simulink model "TST_EISGov_SelectParameter"  (R2016b)
settings: Solver=FixedStepDiscrete  StartTime=0.0  StopTime=simTime  FixedStep=sampleTime  RelTol=1e-3
values from neighbouring files (symbols this model uses):
  testCase = 1    [initTST_EISGov_SelectParameter_001.m]
libraries: simulink x26, UnitTest_Lib x24
(part 2 of 3)

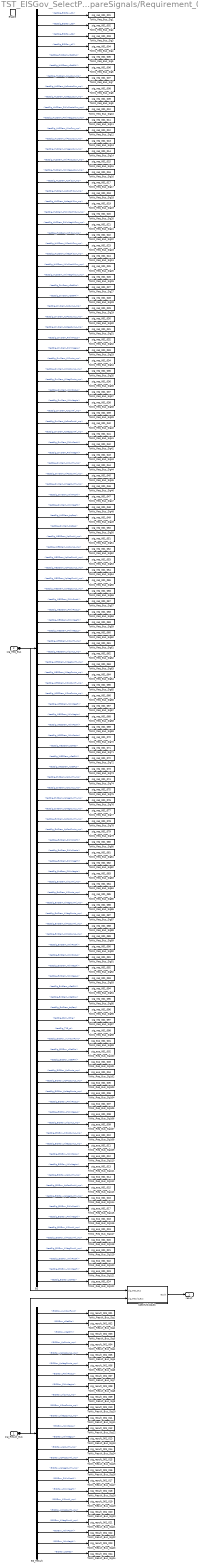
== system TST_EISGov_SelectParameter/compareSignals/Requirement_001 ==
  sig_Result_Bus : Inport
  sig_Req_Bus : Inport  Port=2
  Enable : EnablePort
  BS : BusSelector  OutputSignals=testSig_EISGov_st1,testSig_EISGov_st3,testSig_EISGov_st6,testSig_EISGov_st7,testSig_HLSDem_nSetPLo,testSig_HLSDem_nSetPHi,testSig_HLSDem_KpLoCurr_mp,testSig_HLSDem_KpPosLoCurr_mp,testSig_HLSDem_KpNegLoCurr_mp,testSig_HLSDem_PWinPosLoCurr_mp,testSig_HLSDem_PWinNegLoCurr_mp,testSig_HLSDem_KiLoCurr_mp,testSig_HLSDem_KiPosLoCurr_mp,testSig_HLSDem_KiNegLoCurr_mp,testSig_HLSDem_IWinPosLoCurr_mp,testSig_HLSDem_IWinNegLoCurr_mp,testSig_HLSDem_KpHiCurr_mp,testSig_HLSDem_KpPosHiCurr_mp,testSig_HLSDem_KpNegHiCurr_mp,testSig_HLSDem_PWinPosHiCurr_mp,testSig_HLSDem_PWinNegHiCurr_mp,testSig_HLSDem_KiHiCurr_mp,testSig_HLSDem_KiPosHiCurr_mp,testSig_HLSDem_KiNegHiCurr_mp,testSig_HLSDem_IWinPosHiCurr_mp,testSig_HLSDem_IWinNegHiCurr_mp,testSig_DrvDem_nSetPLo,testSig_DrvDem_nSetPHi,testSig_DrvDem_KpCurrLo_mp,testSig_DrvDem_KpPosCurrLo_mp,testSig_DrvDem_KpNegCurrLo_mp,testSig_DrvDem_PWinPosLo,testSig_DrvDem_PWinNegLo,testSig_DrvDem_KiCurrLo_mp,testSig_DrvDem_KiPosCurrLo_mp,testSig_DrvDem_KiNegCurrLo_mp,testSig_DrvDem_IWinPosLo,testSig_DrvDem_IWinNegLo,testSig_DrvDem_KpCurrHi_mp,testSig_DrvDem_KpPosCurrHi_mp,testSig_DrvDem_KpNegCurrHi_mp,testSig_DrvDem_PWinPosHi,testSig_DrvDem_PWinNegHi,testSig_DrvDem_KiCurrHi_mp,testSig_DrvDem_KiPosCurrHi_mp,testSig_DrvDem_KiNegCurrHi_mp,testSig_DrvDem_IWinPosHi,testSig_DrvDem_IWinNegHi,testSig_HLSDem_trqReq,testSig_DrvDem_trqReq,testSig_WESDem_KpCurrHi_mp,testSig_WESDem_KpCurrLo_mp,testSig_WESDem_KpPosCurrHi_mp,testSig_WESDem_KpPosCurrLo_mp,testSig_WESDem_KpNegCurrHi_mp,testSig_WESDem_KpNegCurrLo_mp,testSig_WESDem_PWinPosHi,testSig_WESDem_PWinPosLo,testSig_WESDem_PWinNegHi,testSig_WESDem_PWinNegLo,testSig_WESDem_KiCurrHi_mp,testSig_WESDem_KiCurrLo_mp,testSig_WESDem_KiNegCurrHi_mp,testSig_WESDem_KiNegCurrLo_mp,testSig_WESDem_KiPosCurrHi_mp,testSig_WESDem_KiPosCurrLo_mp,testSig_WESDem_IWinNegHi,testSig_WESDem_IWinNegLo,testSig_WESDem_IWinPosHi,testSig_WESDem_IWinPosLo,testSig_WESDem_trqReq,testSig_WESDem_nSetPHi,testSig_WESDem_nSetPLo,testSig_ExtDem_KpCurrHi_mp,testSig_ExtDem_KpCurrLo_mp,testSig_ExtDem_KpNegCurrHi_mp,testSig_ExtDem_KpNegCurrLo_mp,testSig_ExtDem_KpPosCurrHi_mp,testSig_ExtDem_KpPosCurrLo_mp,testSig_ExtDem_PWinPosHi,testSig_ExtDem_PWinPosLo,testSig_ExtDem_PWinNegHi,testSig_ExtDem_PWinNegLo,testSig_ExtDem_KiCurrHi_mp,testSig_ExtDem_KiCurrLo_mp,testSig_ExtDem_KiNegCurrHi_mp,testSig_ExtDem_KiNegCurrLo_mp,testSig_ExtDem_KiPosCurrHi_mp,testSig_ExtDem_KiPosCurrLo_mp,testSig_ExtDem_IWinPosHi,testSig_ExtDem_IWinPosLo,testSig_ExtDem_IWinNegHi,testSig_ExtDem_IWinNegLo,testSig_ExtDem_nSetPHi,testSig_ExtDem_nSetPLo,testSig_ExtDem_trqReq,testSig_Epm_nEng,testSig_T15_st,testSig_EISGov_numCurrFunc,testSig_EISGov_nSetPLo,testSig_EISGov_nSetPHi,testSig_EISGov_KpCurrLo_mp,testSig_EISGov_KpPosCurrLo_mp,testSig_EISGov_KpNegCurrLo_mp,testSig_EISGov_PWinPosLo,testSig_EISGov_PWinNegLo,testSig_EISGov_KiCurrLo_mp,testSig_EISGov_KiPosCurrLo_mp,testSig_EISGov_KiNegCurrLo_mp,testSig_EISGov_IWinPosLo,testSig_EISGov_IWinNegLo,testSig_EISGov_KpCurrHi_mp,testSig_EISGov_KpPosCurrHi_mp,testSig_EISGov_KpNegCurrHi_mp,testSig_EISGov_PWinPosHi,testSig_EISGov_PWinNegHi,testSig_EISGov_KiCurrHi_mp,testSig_EISGov_KiPosCurrHi_mp,testSig_EISGov_KiNegCurrHi_mp,testSig_EISGov_IWinPosHi,testSig_EISGov_IWinNegHi,testSig_EISGov_trqReq
  BS_Result : BusSelector  OutputSignals=EISGov_numCurrFunc,EISGov_nSetPLo,EISGov_nSetPHi,EISGov_KpCurrLo_mp,EISGov_KpPosCurrLo_mp,EISGov_KpNegCurrLo_mp,EISGov_PWinPosLo,EISGov_PWinNegLo,EISGov_KiCurrLo_mp,EISGov_KiPosCurrLo_mp,EISGov_KiNegCurrLo_mp,EISGov_IWinPosLo,EISGov_IWinNegLo,EISGov_KpCurrHi_mp,EISGov_KpPosCurrHi_mp,EISGov_KpNegCurrHi_mp,EISGov_PWinPosHi,EISGov_PWinNegHi,EISGov_KiCurrHi_mp,EISGov_KiPosCurrHi_mp,EISGov_KiNegCurrHi_mp,EISGov_IWinPosHi,EISGov_IWinNegHi,EISGov_trqReq
  ToWs_Req_Bus_Sig1 : ToWorkspace  VariableName=sig_req_001_001  SaveFormat=Structure With Time
  ToWs_Req_Bus_Sig10 : ToWorkspace  VariableName=sig_req_001_010  SaveFormat=Structure With Time
  ToWs_Req_Bus_Sig100 : ToWorkspace  VariableName=sig_exp_001_002  SaveFormat=Structure With Time
  ToWs_Req_Bus_Sig101 : ToWorkspace  VariableName=sig_exp_001_003  SaveFormat=Structure With Time
  ToWs_Req_Bus_Sig102 : ToWorkspace  VariableName=sig_exp_001_004  SaveFormat=Structure With Time
  ToWs_Req_Bus_Sig103 : ToWorkspace  VariableName=sig_exp_001_005  SaveFormat=Structure With Time
  ToWs_Req_Bus_Sig104 : ToWorkspace  VariableName=sig_exp_001_006  SaveFormat=Structure With Time
  ToWs_Req_Bus_Sig105 : ToWorkspace  VariableName=sig_exp_001_007  SaveFormat=Structure With Time
  ToWs_Req_Bus_Sig106 : ToWorkspace  VariableName=sig_exp_001_008  SaveFormat=Structure With Time
  ToWs_Req_Bus_Sig107 : ToWorkspace  VariableName=sig_exp_001_009  SaveFormat=Structure With Time
  ToWs_Req_Bus_Sig108 : ToWorkspace  VariableName=sig_exp_001_010  SaveFormat=Structure With Time
  ToWs_Req_Bus_Sig109 : ToWorkspace  VariableName=sig_exp_001_011  SaveFormat=Structure With Time
  ToWs_Req_Bus_Sig11 : ToWorkspace  VariableName=sig_req_001_011  SaveFormat=Structure With Time
  ToWs_Req_Bus_Sig110 : ToWorkspace  VariableName=sig_exp_001_012  SaveFormat=Structure With Time
  ToWs_Req_Bus_Sig111 : ToWorkspace  VariableName=sig_exp_001_013  SaveFormat=Structure With Time
  ToWs_Req_Bus_Sig112 : ToWorkspace  VariableName=sig_exp_001_014  SaveFormat=Structure With Time
  ToWs_Req_Bus_Sig113 : ToWorkspace  VariableName=sig_exp_001_015  SaveFormat=Structure With Time
  ToWs_Req_Bus_Sig114 : ToWorkspace  VariableName=sig_exp_001_016  SaveFormat=Structure With Time
  ToWs_Req_Bus_Sig115 : ToWorkspace  VariableName=sig_exp_001_017  SaveFormat=Structure With Time
  ToWs_Req_Bus_Sig116 : ToWorkspace  VariableName=sig_exp_001_018  SaveFormat=Structure With Time
  ToWs_Req_Bus_Sig117 : ToWorkspace  VariableName=sig_exp_001_019  SaveFormat=Structure With Time
  ToWs_Req_Bus_Sig118 : ToWorkspace  VariableName=sig_exp_001_020  SaveFormat=Structure With Time
  ToWs_Req_Bus_Sig119 : ToWorkspace  VariableName=sig_exp_001_021  SaveFormat=Structure With Time
  ToWs_Req_Bus_Sig12 : ToWorkspace  VariableName=sig_req_001_012  SaveFormat=Structure With Time
  ToWs_Req_Bus_Sig120 : ToWorkspace  VariableName=sig_exp_001_022  SaveFormat=Structure With Time
  ToWs_Req_Bus_Sig121 : ToWorkspace  VariableName=sig_exp_001_023  SaveFormat=Structure With Time
  ToWs_Req_Bus_Sig122 : ToWorkspace  VariableName=sig_exp_001_024  SaveFormat=Structure With Time
  ToWs_Req_Bus_Sig13 : ToWorkspace  VariableName=sig_req_001_013  SaveFormat=Structure With Time
  ToWs_Req_Bus_Sig14 : ToWorkspace  VariableName=sig_req_001_014  SaveFormat=Structure With Time
  ToWs_Req_Bus_Sig15 : ToWorkspace  VariableName=sig_req_001_015  SaveFormat=Structure With Time
  ToWs_Req_Bus_Sig16 : ToWorkspace  VariableName=sig_req_001_016  SaveFormat=Structure With Time
  ToWs_Req_Bus_Sig17 : ToWorkspace  VariableName=sig_req_001_017  SaveFormat=Structure With Time
  ToWs_Req_Bus_Sig18 : ToWorkspace  VariableName=sig_req_001_018  SaveFormat=Structure With Time
  ToWs_Req_Bus_Sig19 : ToWorkspace  VariableName=sig_req_001_019  SaveFormat=Structure With Time
  ToWs_Req_Bus_Sig2 : ToWorkspace  VariableName=sig_req_001_002  SaveFormat=Structure With Time
  ToWs_Req_Bus_Sig20 : ToWorkspace  VariableName=sig_req_001_020  SaveFormat=Structure With Time
  ToWs_Req_Bus_Sig21 : ToWorkspace  VariableName=sig_req_001_021  SaveFormat=Structure With Time
  ToWs_Req_Bus_Sig22 : ToWorkspace  VariableName=sig_req_001_022  SaveFormat=Structure With Time
  ToWs_Req_Bus_Sig23 : ToWorkspace  VariableName=sig_req_001_023  SaveFormat=Structure With Time
  ToWs_Req_Bus_Sig24 : ToWorkspace  VariableName=sig_req_001_024  SaveFormat=Structure With Time
  ToWs_Req_Bus_Sig25 : ToWorkspace  VariableName=sig_req_001_025  SaveFormat=Structure With Time
  ToWs_Req_Bus_Sig26 : ToWorkspace  VariableName=sig_req_001_026  SaveFormat=Structure With Time
  ToWs_Req_Bus_Sig27 : ToWorkspace  VariableName=sig_req_001_027  SaveFormat=Structure With Time
  ToWs_Req_Bus_Sig28 : ToWorkspace  VariableName=sig_req_001_028  SaveFormat=Structure With Time
  ToWs_Req_Bus_Sig29 : ToWorkspace  VariableName=sig_req_001_029  SaveFormat=Structure With Time
  ToWs_Req_Bus_Sig3 : ToWorkspace  VariableName=sig_req_001_003  SaveFormat=Structure With Time
  ToWs_Req_Bus_Sig30 : ToWorkspace  VariableName=sig_req_001_030  SaveFormat=Structure With Time
  ToWs_Req_Bus_Sig31 : ToWorkspace  VariableName=sig_req_001_031  SaveFormat=Structure With Time
  ToWs_Req_Bus_Sig32 : ToWorkspace  VariableName=sig_req_001_032  SaveFormat=Structure With Time
  ToWs_Req_Bus_Sig33 : ToWorkspace  VariableName=sig_req_001_033  SaveFormat=Structure With Time
  ToWs_Req_Bus_Sig34 : ToWorkspace  VariableName=sig_req_001_034  SaveFormat=Structure With Time
  ToWs_Req_Bus_Sig35 : ToWorkspace  VariableName=sig_req_001_035  SaveFormat=Structure With Time
  ToWs_Req_Bus_Sig36 : ToWorkspace  VariableName=sig_req_001_036  SaveFormat=Structure With Time
  ToWs_Req_Bus_Sig37 : ToWorkspace  VariableName=sig_req_001_037  SaveFormat=Structure With Time
  ToWs_Req_Bus_Sig38 : ToWorkspace  VariableName=sig_req_001_038  SaveFormat=Structure With Time
  ToWs_Req_Bus_Sig39 : ToWorkspace  VariableName=sig_req_001_039  SaveFormat=Structure With Time
  ToWs_Req_Bus_Sig4 : ToWorkspace  VariableName=sig_req_001_004  SaveFormat=Structure With Time
  ToWs_Req_Bus_Sig40 : ToWorkspace  VariableName=sig_req_001_040  SaveFormat=Structure With Time
  ToWs_Req_Bus_Sig41 : ToWorkspace  VariableName=sig_req_001_041  SaveFormat=Structure With Time
  ToWs_Req_Bus_Sig42 : ToWorkspace  VariableName=sig_req_001_042  SaveFormat=Structure With Time
  ToWs_Req_Bus_Sig43 : ToWorkspace  VariableName=sig_req_001_043  SaveFormat=Structure With Time
  ToWs_Req_Bus_Sig44 : ToWorkspace  VariableName=sig_req_001_044  SaveFormat=Structure With Time
  ToWs_Req_Bus_Sig45 : ToWorkspace  VariableName=sig_req_001_045  SaveFormat=Structure With Time
  ToWs_Req_Bus_Sig46 : ToWorkspace  VariableName=sig_req_001_046  SaveFormat=Structure With Time
  ToWs_Req_Bus_Sig47 : ToWorkspace  VariableName=sig_req_001_047  SaveFormat=Structure With Time
  ToWs_Req_Bus_Sig48 : ToWorkspace  VariableName=sig_req_001_048  SaveFormat=Structure With Time
  ToWs_Req_Bus_Sig49 : ToWorkspace  VariableName=sig_req_001_049  SaveFormat=Structure With Time
  ToWs_Req_Bus_Sig5 : ToWorkspace  VariableName=sig_req_001_005  SaveFormat=Structure With Time
  ToWs_Req_Bus_Sig50 : ToWorkspace  VariableName=sig_req_001_050  SaveFormat=Structure With Time
  ToWs_Req_Bus_Sig51 : ToWorkspace  VariableName=sig_req_001_051  SaveFormat=Structure With Time
  ToWs_Req_Bus_Sig52 : ToWorkspace  VariableName=sig_req_001_052  SaveFormat=Structure With Time
  ToWs_Req_Bus_Sig53 : ToWorkspace  VariableName=sig_req_001_053  SaveFormat=Structure With Time
  ToWs_Req_Bus_Sig54 : ToWorkspace  VariableName=sig_req_001_054  SaveFormat=Structure With Time
  ToWs_Req_Bus_Sig55 : ToWorkspace  VariableName=sig_req_001_055  SaveFormat=Structure With Time
  ToWs_Req_Bus_Sig56 : ToWorkspace  VariableName=sig_req_001_056  SaveFormat=Structure With Time
  ToWs_Req_Bus_Sig57 : ToWorkspace  VariableName=sig_req_001_057  SaveFormat=Structure With Time
  ToWs_Req_Bus_Sig58 : ToWorkspace  VariableName=sig_req_001_058  SaveFormat=Structure With Time
  ToWs_Req_Bus_Sig59 : ToWorkspace  VariableName=sig_req_001_059  SaveFormat=Structure With Time
  ToWs_Req_Bus_Sig6 : ToWorkspace  VariableName=sig_req_001_006  SaveFormat=Structure With Time
  ToWs_Req_Bus_Sig60 : ToWorkspace  VariableName=sig_req_001_060  SaveFormat=Structure With Time
  ToWs_Req_Bus_Sig61 : ToWorkspace  VariableName=sig_req_001_061  SaveFormat=Structure With Time
  ToWs_Req_Bus_Sig62 : ToWorkspace  VariableName=sig_req_001_062  SaveFormat=Structure With Time
  ToWs_Req_Bus_Sig63 : ToWorkspace  VariableName=sig_req_001_063  SaveFormat=Structure With Time
  ToWs_Req_Bus_Sig64 : ToWorkspace  VariableName=sig_req_001_064  SaveFormat=Structure With Time
  ToWs_Req_Bus_Sig65 : ToWorkspace  VariableName=sig_req_001_065  SaveFormat=Structure With Time
  ToWs_Req_Bus_Sig66 : ToWorkspace  VariableName=sig_req_001_066  SaveFormat=Structure With Time
  ToWs_Req_Bus_Sig67 : ToWorkspace  VariableName=sig_req_001_067  SaveFormat=Structure With Time
  ToWs_Req_Bus_Sig68 : ToWorkspace  VariableName=sig_req_001_068  SaveFormat=Structure With Time
  ToWs_Req_Bus_Sig69 : ToWorkspace  VariableName=sig_req_001_069  SaveFormat=Structure With Time
  ToWs_Req_Bus_Sig7 : ToWorkspace  VariableName=sig_req_001_007  SaveFormat=Structure With Time
  ToWs_Req_Bus_Sig70 : ToWorkspace  VariableName=sig_req_001_070  SaveFormat=Structure With Time
  ToWs_Req_Bus_Sig71 : ToWorkspace  VariableName=sig_req_001_071  SaveFormat=Structure With Time
  ToWs_Req_Bus_Sig72 : ToWorkspace  VariableName=sig_req_001_072  SaveFormat=Structure With Time
  ToWs_Req_Bus_Sig73 : ToWorkspace  VariableName=sig_req_001_073  SaveFormat=Structure With Time
  ToWs_Req_Bus_Sig74 : ToWorkspace  VariableName=sig_req_001_074  SaveFormat=Structure With Time
  ToWs_Req_Bus_Sig75 : ToWorkspace  VariableName=sig_req_001_075  SaveFormat=Structure With Time
  ToWs_Req_Bus_Sig76 : ToWorkspace  VariableName=sig_req_001_076  SaveFormat=Structure With Time
  ToWs_Req_Bus_Sig77 : ToWorkspace  VariableName=sig_req_001_077  SaveFormat=Structure With Time
  ToWs_Req_Bus_Sig78 : ToWorkspace  VariableName=sig_req_001_078  SaveFormat=Structure With Time
  ToWs_Req_Bus_Sig79 : ToWorkspace  VariableName=sig_req_001_079  SaveFormat=Structure With Time
  ToWs_Req_Bus_Sig8 : ToWorkspace  VariableName=sig_req_001_008  SaveFormat=Structure With Time
  ToWs_Req_Bus_Sig80 : ToWorkspace  VariableName=sig_req_001_080  SaveFormat=Structure With Time
  ToWs_Req_Bus_Sig81 : ToWorkspace  VariableName=sig_req_001_081  SaveFormat=Structure With Time
  ToWs_Req_Bus_Sig82 : ToWorkspace  VariableName=sig_req_001_082  SaveFormat=Structure With Time
  ToWs_Req_Bus_Sig83 : ToWorkspace  VariableName=sig_req_001_083  SaveFormat=Structure With Time
  ToWs_Req_Bus_Sig84 : ToWorkspace  VariableName=sig_req_001_084  SaveFormat=Structure With Time
  ToWs_Req_Bus_Sig85 : ToWorkspace  VariableName=sig_req_001_085  SaveFormat=Structure With Time
  ToWs_Req_Bus_Sig86 : ToWorkspace  VariableName=sig_req_001_086  SaveFormat=Structure With Time
  ToWs_Req_Bus_Sig87 : ToWorkspace  VariableName=sig_req_001_087  SaveFormat=Structure With Time
  ToWs_Req_Bus_Sig88 : ToWorkspace  VariableName=sig_req_001_088  SaveFormat=Structure With Time
  ToWs_Req_Bus_Sig89 : ToWorkspace  VariableName=sig_req_001_089  SaveFormat=Structure With Time
  ToWs_Req_Bus_Sig9 : ToWorkspace  VariableName=sig_req_001_009  SaveFormat=Structure With Time
  ToWs_Req_Bus_Sig90 : ToWorkspace  VariableName=sig_req_001_090  SaveFormat=Structure With Time
  ToWs_Req_Bus_Sig91 : ToWorkspace  VariableName=sig_req_001_091  SaveFormat=Structure With Time
  ToWs_Req_Bus_Sig92 : ToWorkspace  VariableName=sig_req_001_092  SaveFormat=Structure With Time
  ToWs_Req_Bus_Sig93 : ToWorkspace  VariableName=sig_req_001_093  SaveFormat=Structure With Time
  ToWs_Req_Bus_Sig94 : ToWorkspace  VariableName=sig_req_001_094  SaveFormat=Structure With Time
  ToWs_Req_Bus_Sig95 : ToWorkspace  VariableName=sig_req_001_095  SaveFormat=Structure With Time
  ToWs_Req_Bus_Sig96 : ToWorkspace  VariableName=sig_req_001_096  SaveFormat=Structure With Time
  ToWs_Req_Bus_Sig97 : ToWorkspace  VariableName=sig_req_001_097  SaveFormat=Structure With Time
  ToWs_Req_Bus_Sig98 : ToWorkspace  VariableName=sig_req_001_098  SaveFormat=Structure With Time
  ToWs_Req_Bus_Sig99 : ToWorkspace  VariableName=sig_exp_001_001  SaveFormat=Structure With Time
  ToWs_Result_Bus_Sig1 : ToWorkspace  VariableName=sig_result_001_001  SaveFormat=Structure With Time
  ToWs_Result_Bus_Sig10 : ToWorkspace  VariableName=sig_result_001_010  SaveFormat=Structure With Time
  ToWs_Result_Bus_Sig11 : ToWorkspace  VariableName=sig_result_001_011  SaveFormat=Structure With Time
  ToWs_Result_Bus_Sig12 : ToWorkspace  VariableName=sig_result_001_012  SaveFormat=Structure With Time
  ToWs_Result_Bus_Sig13 : ToWorkspace  VariableName=sig_result_001_013  SaveFormat=Structure With Time
  ToWs_Result_Bus_Sig14 : ToWorkspace  VariableName=sig_result_001_014  SaveFormat=Structure With Time
  ToWs_Result_Bus_Sig15 : ToWorkspace  VariableName=sig_result_001_015  SaveFormat=Structure With Time
  ToWs_Result_Bus_Sig16 : ToWorkspace  VariableName=sig_result_001_016  SaveFormat=Structure With Time
  ToWs_Result_Bus_Sig17 : ToWorkspace  VariableName=sig_result_001_017  SaveFormat=Structure With Time
  ToWs_Result_Bus_Sig18 : ToWorkspace  VariableName=sig_result_001_018  SaveFormat=Structure With Time
  ToWs_Result_Bus_Sig19 : ToWorkspace  VariableName=sig_result_001_019  SaveFormat=Structure With Time
  ToWs_Result_Bus_Sig2 : ToWorkspace  VariableName=sig_result_001_002  SaveFormat=Structure With Time
  ToWs_Result_Bus_Sig20 : ToWorkspace  VariableName=sig_result_001_020  SaveFormat=Structure With Time
  ToWs_Result_Bus_Sig21 : ToWorkspace  VariableName=sig_result_001_021  SaveFormat=Structure With Time
  ToWs_Result_Bus_Sig22 : ToWorkspace  VariableName=sig_result_001_022  SaveFormat=Structure With Time
  ToWs_Result_Bus_Sig23 : ToWorkspace  VariableName=sig_result_001_023  SaveFormat=Structure With Time
  ToWs_Result_Bus_Sig24 : ToWorkspace  VariableName=sig_result_001_024  SaveFormat=Structure With Time
  ToWs_Result_Bus_Sig3 : ToWorkspace  VariableName=sig_result_001_003  SaveFormat=Structure With Time
  ToWs_Result_Bus_Sig4 : ToWorkspace  VariableName=sig_result_001_004  SaveFormat=Structure With Time
  ToWs_Result_Bus_Sig5 : ToWorkspace  VariableName=sig_result_001_005  SaveFormat=Structure With Time
  ToWs_Result_Bus_Sig6 : ToWorkspace  VariableName=sig_result_001_006  SaveFormat=Structure With Time
  ToWs_Result_Bus_Sig7 : ToWorkspace  VariableName=sig_result_001_007  SaveFormat=Structure With Time
  ToWs_Result_Bus_Sig8 : ToWorkspace  VariableName=sig_result_001_008  SaveFormat=Structure With Time
  ToWs_Result_Bus_Sig9 : ToWorkspace  VariableName=sig_result_001_009  SaveFormat=Structure With Time
  specifyOutputs : Subsystem
  result : Outport
  wires:
  sig_Req_Bus/1 -> BS/1, specifyOutputs/1(sig_Req_Bus)
  BS/1 -> ToWs_Req_Bus_Sig1/1  "<testSig_EISGov_st1>"
  BS/2 -> ToWs_Req_Bus_Sig2/1  "<testSig_EISGov_st3>"
  BS/3 -> ToWs_Req_Bus_Sig3/1  "<testSig_EISGov_st6>"
  BS/4 -> ToWs_Req_Bus_Sig4/1  "<testSig_EISGov_st7>"
  BS/5 -> ToWs_Req_Bus_Sig5/1  "<testSig_HLSDem_nSetPLo>"
  BS/6 -> ToWs_Req_Bus_Sig6/1  "<testSig_HLSDem_nSetPHi>"
  BS/7 -> ToWs_Req_Bus_Sig7/1  "<testSig_HLSDem_KpLoCurr_mp>"
  BS/8 -> ToWs_Req_Bus_Sig8/1  "<testSig_HLSDem_KpPosLoCurr_mp>"
  BS/9 -> ToWs_Req_Bus_Sig9/1  "<testSig_HLSDem_KpNegLoCurr_mp>"
  BS/10 -> ToWs_Req_Bus_Sig10/1  "<testSig_HLSDem_PWinPosLoCurr_mp>"
  BS/11 -> ToWs_Req_Bus_Sig11/1  "<testSig_HLSDem_PWinNegLoCurr_mp>"
  BS/12 -> ToWs_Req_Bus_Sig12/1  "<testSig_HLSDem_KiLoCurr_mp>"
  BS/13 -> ToWs_Req_Bus_Sig13/1  "<testSig_HLSDem_KiPosLoCurr_mp>"
  BS/14 -> ToWs_Req_Bus_Sig14/1  "<testSig_HLSDem_KiNegLoCurr_mp>"
  BS/15 -> ToWs_Req_Bus_Sig15/1  "<testSig_HLSDem_IWinPosLoCurr_mp>"
  BS/16 -> ToWs_Req_Bus_Sig16/1  "<testSig_HLSDem_IWinNegLoCurr_mp>"
  BS/17 -> ToWs_Req_Bus_Sig17/1  "<testSig_HLSDem_KpHiCurr_mp>"
  BS/18 -> ToWs_Req_Bus_Sig18/1  "<testSig_HLSDem_KpPosHiCurr_mp>"
  BS/19 -> ToWs_Req_Bus_Sig19/1  "<testSig_HLSDem_KpNegHiCurr_mp>"
  BS/20 -> ToWs_Req_Bus_Sig20/1  "<testSig_HLSDem_PWinPosHiCurr_mp>"
  BS/21 -> ToWs_Req_Bus_Sig21/1  "<testSig_HLSDem_PWinNegHiCurr_mp>"
  BS/22 -> ToWs_Req_Bus_Sig22/1  "<testSig_HLSDem_KiHiCurr_mp>"
  BS/23 -> ToWs_Req_Bus_Sig23/1  "<testSig_HLSDem_KiPosHiCurr_mp>"
  BS/24 -> ToWs_Req_Bus_Sig24/1  "<testSig_HLSDem_KiNegHiCurr_mp>"
  BS/25 -> ToWs_Req_Bus_Sig25/1  "<testSig_HLSDem_IWinPosHiCurr_mp>"
  BS/26 -> ToWs_Req_Bus_Sig26/1  "<testSig_HLSDem_IWinNegHiCurr_mp>"
  BS/27 -> ToWs_Req_Bus_Sig27/1  "<testSig_DrvDem_nSetPLo>"
  BS/28 -> ToWs_Req_Bus_Sig28/1  "<testSig_DrvDem_nSetPHi>"
  BS/29 -> ToWs_Req_Bus_Sig29/1  "<testSig_DrvDem_KpCurrLo_mp>"
  BS/30 -> ToWs_Req_Bus_Sig30/1  "<testSig_DrvDem_KpPosCurrLo_mp>"
  BS/31 -> ToWs_Req_Bus_Sig31/1  "<testSig_DrvDem_KpNegCurrLo_mp>"
  BS/32 -> ToWs_Req_Bus_Sig32/1  "<testSig_DrvDem_PWinPosLo>"
  BS/33 -> ToWs_Req_Bus_Sig33/1  "<testSig_DrvDem_PWinNegLo>"
  BS/34 -> ToWs_Req_Bus_Sig34/1  "<testSig_DrvDem_KiCurrLo_mp>"
  BS/35 -> ToWs_Req_Bus_Sig35/1  "<testSig_DrvDem_KiPosCurrLo_mp>"
  BS/36 -> ToWs_Req_Bus_Sig36/1  "<testSig_DrvDem_KiNegCurrLo_mp>"
  BS/37 -> ToWs_Req_Bus_Sig37/1  "<testSig_DrvDem_IWinPosLo>"
  BS/38 -> ToWs_Req_Bus_Sig38/1  "<testSig_DrvDem_IWinNegLo>"
  BS/39 -> ToWs_Req_Bus_Sig39/1  "<testSig_DrvDem_KpCurrHi_mp>"
  BS/40 -> ToWs_Req_Bus_Sig40/1  "<testSig_DrvDem_KpPosCurrHi_mp>"
  BS/41 -> ToWs_Req_Bus_Sig41/1  "<testSig_DrvDem_KpNegCurrHi_mp>"
  BS/42 -> ToWs_Req_Bus_Sig42/1  "<testSig_DrvDem_PWinPosHi>"
  BS/43 -> ToWs_Req_Bus_Sig43/1  "<testSig_DrvDem_PWinNegHi>"
  BS/44 -> ToWs_Req_Bus_Sig44/1  "<testSig_DrvDem_KiCurrHi_mp>"
  BS/45 -> ToWs_Req_Bus_Sig45/1  "<testSig_DrvDem_KiPosCurrHi_mp>"
  BS/46 -> ToWs_Req_Bus_Sig46/1  "<testSig_DrvDem_KiNegCurrHi_mp>"
  BS/47 -> ToWs_Req_Bus_Sig47/1  "<testSig_DrvDem_IWinPosHi>"
  BS/48 -> ToWs_Req_Bus_Sig48/1  "<testSig_DrvDem_IWinNegHi>"
  BS/49 -> ToWs_Req_Bus_Sig49/1  "<testSig_HLSDem_trqReq>"
  BS/50 -> ToWs_Req_Bus_Sig50/1  "<testSig_DrvDem_trqReq>"
  BS/51 -> ToWs_Req_Bus_Sig51/1  "<testSig_WESDem_KpCurrHi_mp>"
  BS/52 -> ToWs_Req_Bus_Sig52/1  "<testSig_WESDem_KpCurrLo_mp>"
  BS/53 -> ToWs_Req_Bus_Sig53/1  "<testSig_WESDem_KpPosCurrHi_mp>"
  BS/54 -> ToWs_Req_Bus_Sig54/1  "<testSig_WESDem_KpPosCurrLo_mp>"
  BS/55 -> ToWs_Req_Bus_Sig55/1  "<testSig_WESDem_KpNegCurrHi_mp>"
  BS/56 -> ToWs_Req_Bus_Sig56/1  "<testSig_WESDem_KpNegCurrLo_mp>"
  BS/57 -> ToWs_Req_Bus_Sig57/1  "<testSig_WESDem_PWinPosHi>"
  BS/58 -> ToWs_Req_Bus_Sig58/1  "<testSig_WESDem_PWinPosLo>"
  BS/59 -> ToWs_Req_Bus_Sig59/1  "<testSig_WESDem_PWinNegHi>"
  BS/60 -> ToWs_Req_Bus_Sig60/1  "<testSig_WESDem_PWinNegLo>"
  BS/61 -> ToWs_Req_Bus_Sig61/1  "<testSig_WESDem_KiCurrHi_mp>"
  BS/62 -> ToWs_Req_Bus_Sig62/1  "<testSig_WESDem_KiCurrLo_mp>"
  BS/63 -> ToWs_Req_Bus_Sig63/1  "<testSig_WESDem_KiNegCurrHi_mp>"
  BS/64 -> ToWs_Req_Bus_Sig64/1  "<testSig_WESDem_KiNegCurrLo_mp>"
  BS/65 -> ToWs_Req_Bus_Sig65/1  "<testSig_WESDem_KiPosCurrHi_mp>"
  BS/66 -> ToWs_Req_Bus_Sig66/1  "<testSig_WESDem_KiPosCurrLo_mp>"
  BS/67 -> ToWs_Req_Bus_Sig67/1  "<testSig_WESDem_IWinNegHi>"
  BS/68 -> ToWs_Req_Bus_Sig68/1  "<testSig_WESDem_IWinNegLo>"
  BS/69 -> ToWs_Req_Bus_Sig69/1  "<testSig_WESDem_IWinPosHi>"
  BS/70 -> ToWs_Req_Bus_Sig70/1  "<testSig_WESDem_IWinPosLo>"
  BS/71 -> ToWs_Req_Bus_Sig71/1  "<testSig_WESDem_trqReq>"
  BS/72 -> ToWs_Req_Bus_Sig72/1  "<testSig_WESDem_nSetPHi>"
  BS/73 -> ToWs_Req_Bus_Sig73/1  "<testSig_WESDem_nSetPLo>"
  BS/74 -> ToWs_Req_Bus_Sig74/1  "<testSig_ExtDem_KpCurrHi_mp>"
  BS/75 -> ToWs_Req_Bus_Sig75/1  "<testSig_ExtDem_KpCurrLo_mp>"
  BS/76 -> ToWs_Req_Bus_Sig76/1  "<testSig_ExtDem_KpNegCurrHi_mp>"
  BS/77 -> ToWs_Req_Bus_Sig77/1  "<testSig_ExtDem_KpNegCurrLo_mp>"
  BS/78 -> ToWs_Req_Bus_Sig78/1  "<testSig_ExtDem_KpPosCurrHi_mp>"
  BS/79 -> ToWs_Req_Bus_Sig79/1  "<testSig_ExtDem_KpPosCurrLo_mp>"
  BS/80 -> ToWs_Req_Bus_Sig80/1  "<testSig_ExtDem_PWinPosHi>"
  BS/81 -> ToWs_Req_Bus_Sig81/1  "<testSig_ExtDem_PWinPosLo>"
  BS/82 -> ToWs_Req_Bus_Sig82/1  "<testSig_ExtDem_PWinNegHi>"
  BS/83 -> ToWs_Req_Bus_Sig83/1  "<testSig_ExtDem_PWinNegLo>"
  BS/84 -> ToWs_Req_Bus_Sig84/1  "<testSig_ExtDem_KiCurrHi_mp>"
  BS/85 -> ToWs_Req_Bus_Sig85/1  "<testSig_ExtDem_KiCurrLo_mp>"
  BS/86 -> ToWs_Req_Bus_Sig86/1  "<testSig_ExtDem_KiNegCurrHi_mp>"
  BS/87 -> ToWs_Req_Bus_Sig87/1  "<testSig_ExtDem_KiNegCurrLo_mp>"
  BS/88 -> ToWs_Req_Bus_Sig88/1  "<testSig_ExtDem_KiPosCurrHi_mp>"
  BS/89 -> ToWs_Req_Bus_Sig89/1  "<testSig_ExtDem_KiPosCurrLo_mp>"
  BS/90 -> ToWs_Req_Bus_Sig90/1  "<testSig_ExtDem_IWinPosHi>"
  BS/91 -> ToWs_Req_Bus_Sig91/1  "<testSig_ExtDem_IWinPosLo>"
  BS/92 -> ToWs_Req_Bus_Sig92/1  "<testSig_ExtDem_IWinNegHi>"
  BS/93 -> ToWs_Req_Bus_Sig93/1  "<testSig_ExtDem_IWinNegLo>"
  BS/94 -> ToWs_Req_Bus_Sig94/1  "<testSig_ExtDem_nSetPHi>"
  BS/95 -> ToWs_Req_Bus_Sig95/1  "<testSig_ExtDem_nSetPLo>"
  BS/96 -> ToWs_Req_Bus_Sig96/1  "<testSig_ExtDem_trqReq>"
  BS/97 -> ToWs_Req_Bus_Sig97/1  "<testSig_Epm_nEng>"
  BS/98 -> ToWs_Req_Bus_Sig98/1  "<testSig_T15_st>"
  BS/99 -> ToWs_Req_Bus_Sig99/1  "<testSig_EISGov_numCurrFunc>"
  BS/100 -> ToWs_Req_Bus_Sig100/1  "<testSig_EISGov_nSetPLo>"
  BS/101 -> ToWs_Req_Bus_Sig101/1  "<testSig_EISGov_nSetPHi>"
  BS/102 -> ToWs_Req_Bus_Sig102/1  "<testSig_EISGov_KpCurrLo_mp>"
  BS/103 -> ToWs_Req_Bus_Sig103/1  "<testSig_EISGov_KpPosCurrLo_mp>"
  BS/104 -> ToWs_Req_Bus_Sig104/1  "<testSig_EISGov_KpNegCurrLo_mp>"
  BS/105 -> ToWs_Req_Bus_Sig105/1  "<testSig_EISGov_PWinPosLo>"
  BS/106 -> ToWs_Req_Bus_Sig106/1  "<testSig_EISGov_PWinNegLo>"
  BS/107 -> ToWs_Req_Bus_Sig107/1  "<testSig_EISGov_KiCurrLo_mp>"
  BS/108 -> ToWs_Req_Bus_Sig108/1  "<testSig_EISGov_KiPosCurrLo_mp>"
  BS/109 -> ToWs_Req_Bus_Sig109/1  "<testSig_EISGov_KiNegCurrLo_mp>"
  BS/110 -> ToWs_Req_Bus_Sig110/1  "<testSig_EISGov_IWinPosLo>"
  BS/111 -> ToWs_Req_Bus_Sig111/1  "<testSig_EISGov_IWinNegLo>"
  BS/112 -> ToWs_Req_Bus_Sig112/1  "<testSig_EISGov_KpCurrHi_mp>"
  BS/113 -> ToWs_Req_Bus_Sig113/1  "<testSig_EISGov_KpPosCurrHi_mp>"
  BS/114 -> ToWs_Req_Bus_Sig114/1  "<testSig_EISGov_KpNegCurrHi_mp>"
  BS/115 -> ToWs_Req_Bus_Sig115/1  "<testSig_EISGov_PWinPosHi>"
  BS/116 -> ToWs_Req_Bus_Sig116/1  "<testSig_EISGov_PWinNegHi>"
  BS/117 -> ToWs_Req_Bus_Sig117/1  "<testSig_EISGov_KiCurrHi_mp>"
  BS/118 -> ToWs_Req_Bus_Sig118/1  "<testSig_EISGov_KiPosCurrHi_mp>"
  BS/119 -> ToWs_Req_Bus_Sig119/1  "<testSig_EISGov_KiNegCurrHi_mp>"
  BS/120 -> ToWs_Req_Bus_Sig120/1  "<testSig_EISGov_IWinPosHi>"
  BS/121 -> ToWs_Req_Bus_Sig121/1  "<testSig_EISGov_IWinNegHi>"
  BS/122 -> ToWs_Req_Bus_Sig122/1  "<testSig_EISGov_trqReq>"
  sig_Result_Bus/1 -> BS_Result/1, specifyOutputs/2(sig_Result_Bus)
  BS_Result/1 -> ToWs_Result_Bus_Sig1/1  "<EISGov_numCurrFunc>"
  BS_Result/2 -> ToWs_Result_Bus_Sig2/1  "<EISGov_nSetPLo>"
  BS_Result/3 -> ToWs_Result_Bus_Sig3/1  "<EISGov_nSetPHi>"
  BS_Result/4 -> ToWs_Result_Bus_Sig4/1  "<EISGov_KpCurrLo_mp>"
  BS_Result/5 -> ToWs_Result_Bus_Sig5/1  "<EISGov_KpPosCurrLo_mp>"
  BS_Result/6 -> ToWs_Result_Bus_Sig6/1  "<EISGov_KpNegCurrLo_mp>"
  BS_Result/7 -> ToWs_Result_Bus_Sig7/1  "<EISGov_PWinPosLo>"
  BS_Result/8 -> ToWs_Result_Bus_Sig8/1  "<EISGov_PWinNegLo>"
  BS_Result/9 -> ToWs_Result_Bus_Sig9/1  "<EISGov_KiCurrLo_mp>"
  BS_Result/10 -> ToWs_Result_Bus_Sig10/1  "<EISGov_KiPosCurrLo_mp>"
  BS_Result/11 -> ToWs_Result_Bus_Sig11/1  "<EISGov_KiNegCurrLo_mp>"
  BS_Result/12 -> ToWs_Result_Bus_Sig12/1  "<EISGov_IWinPosLo>"
  BS_Result/13 -> ToWs_Result_Bus_Sig13/1  "<EISGov_IWinNegLo>"
  BS_Result/14 -> ToWs_Result_Bus_Sig14/1  "<EISGov_KpCurrHi_mp>"
  BS_Result/15 -> ToWs_Result_Bus_Sig15/1  "<EISGov_KpPosCurrHi_mp>"
  BS_Result/16 -> ToWs_Result_Bus_Sig16/1  "<EISGov_KpNegCurrHi_mp>"
  BS_Result/17 -> ToWs_Result_Bus_Sig17/1  "<EISGov_PWinPosHi>"
  BS_Result/18 -> ToWs_Result_Bus_Sig18/1  "<EISGov_PWinNegHi>"
  BS_Result/19 -> ToWs_Result_Bus_Sig19/1  "<EISGov_KiCurrHi_mp>"
  BS_Result/20 -> ToWs_Result_Bus_Sig20/1  "<EISGov_KiPosCurrHi_mp>"
  BS_Result/21 -> ToWs_Result_Bus_Sig21/1  "<EISGov_KiNegCurrHi_mp>"
  BS_Result/22 -> ToWs_Result_Bus_Sig22/1  "<EISGov_IWinPosHi>"
  BS_Result/23 -> ToWs_Result_Bus_Sig23/1  "<EISGov_IWinNegHi>"
  BS_Result/24 -> ToWs_Result_Bus_Sig24/1  "<EISGov_trqReq>"
  specifyOutputs/1(result) -> result/1
